simulink model "DFT1"  (R2020a)
settings: Solver=VariableStepAuto  StartTime=0.0  StopTime=10.0  RelTol=1e-3
settings Model: Creator=User  LastModifiedBy=User

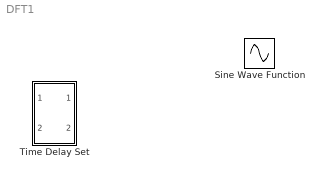
== system DFT1 ==
  Sine Wave Function : Sin  TimeSource=Use external signal  SampleTime=0
  Time Delay Set : Subsystem

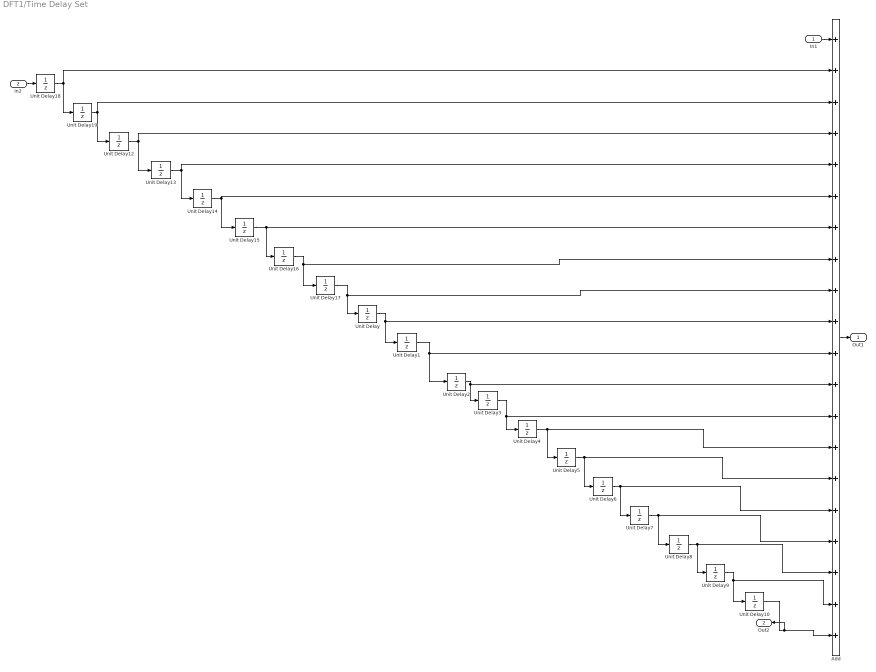
== system DFT1/Time Delay Set ==
  In1 : Inport
  In2 : Inport  Port=2
  Add : Sum  Inputs=++++++++++++++++++++
  Unit Delay{,1..10,12..19} (19 alike) : UnitDelay  SampleTime=-1  HasFrameUpgradeWarning=on
  Out1 : Outport
  Out2 : Outport  Port=2
  wires:
  Unit Delay7/1 -> Unit Delay8/1, Add/17
  In1/1 -> Add/1
  Unit Delay5/1 -> Unit Delay6/1, Add/15
  Unit Delay9/1 -> Unit Delay10/1, Add/19
  Unit Delay16/1 -> Unit Delay17/1, Add/8
  Add/1 -> Out1/1
  Unit Delay15/1 -> Unit Delay16/1, Add/7
  Unit Delay13/1 -> Unit Delay14/1, Add/5
  Unit Delay1/1 -> Unit Delay2/1, Add/11
  Unit Delay3/1 -> Unit Delay4/1, Add/13
  Unit Delay12/1 -> Unit Delay13/1, Add/4
  Unit Delay2/1 -> Add/12, Unit Delay3/1
  Unit Delay17/1 -> Unit Delay/1, Add/9
  Unit Delay10/1 -> Out2/1, Add/20
  Unit Delay4/1 -> Unit Delay5/1, Add/14
  Unit Delay14/1 -> Unit Delay15/1, Add/6
  Unit Delay6/1 -> Unit Delay7/1, Add/16
  Unit Delay/1 -> Unit Delay1/1, Add/10
  Unit Delay18/1 -> Add/2, Unit Delay19/1
  Unit Delay8/1 -> Unit Delay9/1, Add/18
  Unit Delay19/1 -> Add/3, Unit Delay12/1
  In2/1 -> Unit Delay18/1
